simulink model "BEVplantModel"  (R2022b)
settings: Solver=daessc  StartTime=0  StopTime=50  RelTol=1e-3
PreLoadFcn:
  | % Load all parameters
  | BEVplantModelParam;
undefined symbols (not defined in the file): battery, cabin_T_init, coolant_pipe_D, coolant_valve_D_ratio_max, coolant_valve_D_ratio_min, coolant_valve_displacement, electricDrive, max_torque, vehicle, vehicleThermal
libraries: fl_lib x292, nesl_utility x67, SimscapeFluids_lib x15, ee_lib x11, sdl_lib x8, BatteryCurrentManagement x3, slpidlib x3, simulink x2, BatteryThermalManagement x1, autolibshared x1
(part 7 of 10)

== system BEVplantModel/Controller/BMS/MinMax Current Limiter/ODprotection ==
  Cur : Inport
  VoltMin : Inport  Port=2
  CellTpMax : Inport  Port=3
  CellTpMin : Inport  Port=4
  Add : Sum  Inputs=-+
  Constant : Constant  Value=10
  DchrgCurLim : Gain  Gain=battery.MaxDchrgCurLim
  DischCurrLimitMaxTp : Lookup_n-D  NumberOfTableDimensions=1  BreakpointsForDimension1=single([313, 318, 323, 333])  BreakpointsForDimension3=[5, 7]  Table=single([1, 0.5, 0.3, 0])  ExtrapMethod=Clip  UseLastTableValue=on  InternalRulePriority=Speed  RndMeth=Simplest
  DischCurrLimitMinTp : Lookup_n-D  NumberOfTableDimensions=1  BreakpointsForDimension1="single([263, 268,    273,   278, 283, 288, 293])"  BreakpointsForDimension3=[5, 7]  Table="single([0,  0.2, 0.3, 0.5, 0.75, 1, 1])"  ExtrapMethod=Clip  UseLastTableValue=on  InternalRulePriority=Speed  RndMeth=Simplest
  DischCurrLimitVolt : Lookup_n-D  NumberOfTableDimensions=1  BreakpointsForDimension1=single([2.5;3;3.5;4.2])  BreakpointsForDimension3=[5, 7]  Table=single([0 0.25 0.5 0.75])  ExtrapMethod=Clip  UseLastTableValue=on  InternalRulePriority=Speed  RndMeth=Simplest
  Gain : Gain  Gain=2
  Min : MinMax  Inputs=3
  Np_Module : Gain  Gain=battery.Np
  Relational Operator : RelationalOperator  Operator=<=  OutDataTypeStr=boolean  RndMeth=Simplest  InputSameDT=off
  DschCurLim : Outport
  ODWarn : Outport  Port=2
  tag scope: DschCurLim=global
  wires:
  Constant/1 -> Add/1
  Add/1 -> Relational Operator/1
  Relational Operator/1 -> ODWarn/1
  [DschCurLim] -> Add/2
  Cur/1 -> Relational Operator/2
  Min/1 -> DchrgCurLim/1
  DischCurrLimitMinTp/1 -> Min/3  "DischCurrLimMinTp"
  DischCurrLimitMaxTp/1 -> Min/2  "DischCurrLimMaxTp"
  CellTpMax/1 -> DischCurrLimitMaxTp/1
  Np_Module/1 -> [DschCurLim], Gain/1  "CurDchLmt"
  DchrgCurLim/1 -> Np_Module/1
  DischCurrLimitVolt/1 -> Min/1  "DischCurrLimVolt"
  VoltMin/1 -> DischCurrLimitVolt/1
  CellTpMin/1 -> DischCurrLimitMinTp/1
  Gain/1 -> DschCurLim/1  "CurDchLmt"

== system BEVplantModel/Controller/Range Estimator/Online Range/Energy Consumption ==
  V : Inport
  I : Inport  Port=2
  Constant : Constant  Value=3600
  Divide : Product  Inputs=*/
  Gain : Gain  Gain=-1
  Integrator : Integrator
  Product : Product
  E : Outport
  wires:
  Gain/1 -> Product/2
  Constant/1 -> Divide/2
  Integrator/1 -> Divide/1
  Product/1 -> Integrator/1
  I/1 -> Gain/1
  V/1 -> Product/1
  Divide/1 -> E/1

== system BEVplantModel/Controller/Range Estimator/Online Range/Subsystem ==
  E : Inport
  d : Inport  Port=2
  Add : Sum
  Constant2 : Constant
  Divide2 : Product  Inputs=*/
  E/D : Outport
  wires:
  Add/1 -> E/D/1
  Constant2/1 -> Add/2
  Divide2/1 -> Add/1
  d/1 -> Divide2/2
  E/1 -> Divide2/1

== system BEVplantModel/Controller/Thermal Control/Coolant Control/Battery Heater ==
  T_env : Inport
  T_coolant_battery_in : Inport  Port=2
  Constant : Constant  Value=0
  Relay : Relay  OnSwitchValue=15+273.15  OffSwitchValue=5+273.15  OnOutputValue=0  OffOutputValue=1  ZeroCross=off
  Switch : Switch  Criteria=u2 > Threshold  Threshold=5+273.15  SaturateOnIntegerOverflow=off  InputSameDT=off
  cmd_heater : Outport
  wires:
  Constant/1 -> Switch/1
  Relay/1 -> Switch/3
  T_env/1 -> Switch/2
  Switch/1 -> cmd_heater/1
  T_coolant_battery_in/1 -> Relay/1

== system BEVplantModel/Controller/Thermal Control/Coolant Control/Battery Pump ==
  cmd_motor_pump : Inport
  T_battery : Inport  Port=2
  cmd_chiller_bypass : Inport  Port=3
  parallel_serial : Inport  Port=4
  Constant : Constant  Value=0.3
  Constant1 : Constant  Value=0.5
  MinMax : MinMax  Function=max  Inputs=2
  Relay : Relay  OnSwitchValue=50+273.15  OffSwitchValue=45+273.15
  Switch : Switch  Criteria=u2 > Threshold  Threshold=0.5  SaturateOnIntegerOverflow=off  InputSameDT=off
  Switch1 : Switch  Criteria=u2 > Threshold  Threshold=0.5  SaturateOnIntegerOverflow=off  InputSameDT=off
  cmd_battery_pump : Outport
  wires:
  cmd_motor_pump/1 -> Switch/1
  MinMax/1 -> Switch/3
  Switch1/1 -> MinMax/2
  Relay/1 -> MinMax/1
  cmd_chiller_bypass/1 -> Switch1/2
  Constant1/1 -> Switch1/3
  Constant/1 -> Switch1/1
  Switch/1 -> cmd_battery_pump/1
  parallel_serial/1 -> Switch/2
  T_battery/1 -> Relay/1

== system BEVplantModel/Controller/Thermal Control/Coolant Control/Chiller Bypass ==
  T_battery : Inport
  Relay : Relay  OnSwitchValue=35+273.15  OffSwitchValue=30+273.15  OnOutputValue=0  OffOutputValue=1
  cmd_chiller_bypass : Outport
  wires:
  T_battery/1 -> Relay/1
  Relay/1 -> cmd_chiller_bypass/1

== system BEVplantModel/Controller/Thermal Control/Coolant Control/Motor Pump ==
  T_motor : Inport
  1-D Lookup Table : Lookup_n-D  NumberOfTableDimensions=1  BreakpointsForDimension1=[223.15 318.15 321.15 325.15 331.15 333.15 348.15 403.15]  IndexSearchMethod=Linear search  BeginIndexSearchUsingPreviousIndexResult=on  Table=[0 0 0.1 0.3 0.5 0.7 1 1]  InternalRulePriority=Speed  RndMeth=Simplest
  Saturation : Saturate  UpperLimit=1  LowerLimit=0.3
  cmd_motor_pump : Outport
  wires:
  Saturation/1 -> cmd_motor_pump/1
  1-D Lookup Table/1 -> Saturation/1
  T_motor/1 -> 1-D Lookup Table/1

== system BEVplantModel/Controller/Thermal Control/Coolant Control/Parallel-Serial Mode ==
  note: 0 = Parallel mode
      |
      | 1 = Serial mode
  cmd_chiller_bypass : Inport
  T_env : Inport  Port=2
  T_coolant_motor_out : Inport  Port=3
  Constant : Constant  Value=0
  MinMax : MinMax  Function=max  Inputs=2
  Relay : Relay  OnSwitchValue=35+273.15  OffSwitchValue=30+273.15  OnOutputValue=0  OffOutputValue=1
  Switch : Switch  Criteria=u2 > Threshold  Threshold=0.5  SaturateOnIntegerOverflow=off  InputSameDT=off
  cmd_parallel_serial : Outport
  wires:
  Relay/1 -> Switch/1
  cmd_chiller_bypass/1 -> Switch/2
  Switch/1 -> cmd_parallel_serial/1
  Constant/1 -> Switch/3
  MinMax/1 -> Relay/1
  T_coolant_motor_out/1 -> MinMax/2
  T_env/1 -> MinMax/1

== system BEVplantModel/Controller/Thermal Control/Coolant Control/Radiator Bypass ==
  T_coolant_motor_out : Inport
  Relay : Relay  OnSwitchValue=25+273.15  OffSwitchValue=20+273.15  OnOutputValue=0  OffOutputValue=1
  cmd_rad_bypass : Outport
  wires:
  T_coolant_motor_out/1 -> Relay/1
  Relay/1 -> cmd_rad_bypass/1

== system BEVplantModel/Controller/Thermal Control/Fan Control/Motor Requirement ==
  T_motor : Inport
  1-D Lookup Table : Lookup_n-D  NumberOfTableDimensions=1  BreakpointsForDimension1=[223.15 318.15 321.15 325.15 331.15 333.15 348.15 403.15]  IndexSearchMethod=Linear search  BeginIndexSearchUsingPreviousIndexResult=on  Table=[0 0 0.1 0.3 0.5 0.7 1 1]  InternalRulePriority=Speed  RndMeth=Simplest
  cmd_fan : Outport
  wires:
  1-D Lookup Table/1 -> cmd_fan/1
  T_motor/1 -> 1-D Lookup Table/1

== system BEVplantModel/Controller/Vehicle Control/Driver/Motor Speed Reference ==
  VehSpd : Inport  Unit=km/hr
  Constant1 : Constant  Value=vehicle.tireRollingRadius_cm
  Constant2 : Constant  Value=10/3
  Divide : Product  Inputs=*/
  Gain : Gain  Gain=2*pi
  Gain1 : Gain  Gain=1/100
  Product : Product
  Signal Specification : SignalSpecification  Unit=m/min
  Unit Conversion : UnitConversion
  MotorSpdRef : Outport  Unit=rpm  VectorParamsAs1DForOutWhenUnconnected=off
  wires:
  VehSpd/1 -> Unit Conversion/1
  Unit Conversion/1 -> Signal Specification/1
  Signal Specification/1 -> Divide/1
  Constant1/1 -> Gain1/1  "cm"
  Gain/1 -> Divide/2  "2*pi*R (m)"
  Divide/1 -> Product/1  "tireRpmRef"
  Constant2/1 -> Product/2
  Product/1 -> MotorSpdRef/1  "motorRpmRef"
  Gain1/1 -> Gain/1  "m"

== system BEVplantModel/Controller/Vehicle Control/Driver/Speed Controller ==
  Spd : Inport  Unit=rpm
      settings: AttributesFormatString=%<Unit>
  SpdRef : Inport  Port=2  Unit=rpm
      settings: AttributesFormatString=%<Unit>
  20Hz Lowpass Filter : TransferFcn  Denominator=[1/(2*pi*20) 1]
  Constant : Constant  Value=0
  GreaterThan : RelationalOperator  Operator=>  OutDataTypeStr=boolean  RndMeth=Simplest  InputSameDT=off
  Ki : Gain  Gain=5
  Kp : Gain  Gain=5
  Limits [-40,40] : Integrator  ExternalReset=rising  LimitOutput=on  UpperSaturationLimit=40  LowerSaturationLimit=-40  ZeroCross=off
  Saturation : Saturate  UpperLimit=vehicle.motorDrive.simplePmsmDrv_trqMax_Nm  LowerLimit=-vehicle.motorDrive.simplePmsmDrv_trqMax_Nm
      settings: AttributesFormatString=|
      | %<UpperLimit>
      | %<LowerLimit>
  Sum : Sum  Inputs=-+|
  Sum1 : Sum  Inputs=++|
  TrqPID : Outport  Unit=N*m  VectorParamsAs1DForOutWhenUnconnected=off
      settings: AttributesFormatString=%<Unit>
  wires:
  Saturation/1 -> TrqPID/1
  20Hz Lowpass Filter/1 -> GreaterThan/2, Sum/1
  Limits [-40,40]/1 -> Sum1/1
  Kp/1 -> Sum1/2
  Ki/1 -> Limits [-40,40]/1
  Sum/1 -> Kp/1, Ki/1
  Sum1/1 -> Saturation/1
  Spd/1 -> 20Hz Lowpass Filter/1
  SpdRef/1 -> Sum/2
  Constant/1 -> GreaterThan/1
  GreaterThan/1 -> Limits [-40,40]/2

== system BEVplantModel/Controller/Vehicle Control/Torque Control/Brake//Motor Trq Split ==
  note: Torque split between Break model and Modtor drive.
      | TrqCmdPID=Break torque + motor Torque
  TrqReq : Inport
  TrqLimit : Inport  Port=2
  BreakOn : Inport  Port=3
  Abs : Abs  ZeroCross=off  SaturateOnIntegerOverflow=off
  Braking Torque : Subsystem
  Bus Selector : BusSelector  OutputSignals=MaxChrgTrq,MaxDchTorque
  Constant : Constant  Value=vehicle.BrakeFactor
  Max1 : MinMax  Inputs=2  ZeroCross=off
  Switch : Switch  Criteria=u2 > Threshold  SaturateOnIntegerOverflow=off  InputSameDT=off
  TorqueCmd : Outport
  BrkTrq : Outport  Port=2
  wires:
  Bus Selector/2 -> Max1/1  "<MaxDchTorque>"
  TrqReq/1 -> Max1/2
  BreakOn/1 -> Switch/2
  Max1/1 -> Braking Torque/3(BrkTq), Switch/3
  TrqLimit/1 -> Bus Selector/1
  Braking Torque/1(MechBrkTq) -> Abs/1
  Braking Torque/2(RegenBrkTq) -> Switch/1
  Switch/1 -> TorqueCmd/1
  Abs/1 -> BrkTrq/1
  Bus Selector/1 -> Braking Torque/2(MaxChgTq)  "<MaxChrgTrq>"
  Constant/1 -> Braking Torque/1(BrkFac)

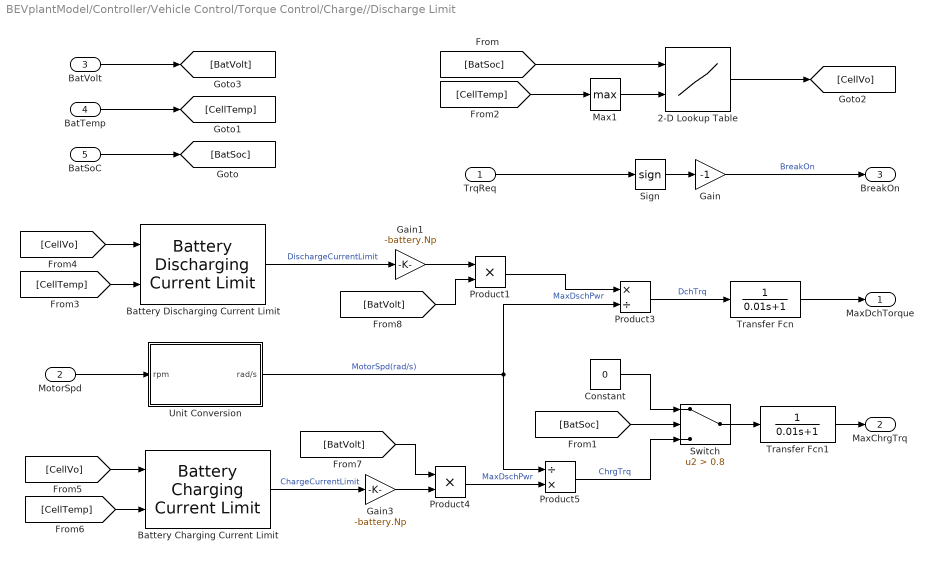
== system BEVplantModel/Controller/Vehicle Control/Torque Control/Charge//Discharge Limit ==
  TrqReq : Inport
  MotorSpd : Inport  Port=2
  BatVolt : Inport  Port=3
  BatTemp : Inport  Port=4
  BatSoC : Inport  Port=5
  2-D Lookup Table : Lookup_n-D  BreakpointsForDimension1=battery.SOC_vec  BreakpointsForDimension2=battery.T_vec  Table=battery.V0_mat  InternalRulePriority=Speed  RndMeth=Simplest
      settings: InputPortMap=u0,u1
  Battery Charging Current Limit : BatteryCurrentManagement/Battery Charging Current Limit  CellOvervoltageLimit=4.5  R0=0.0025  T_vec=[243.15, 258.15, 273.15, 288.15, 303.15, 318.15, 333.15]  CurrentLimitCoolestCell=[ 0, 0,0.5* battery.AH, battery.AH, battery.AH, battery.AH, battery.AH]  CurrentLimitHottestCell="[ battery.AH,  battery.AH,  battery.AH,  battery.AH,  battery.AH,  0.5*battery.AH, 0]"
      settings: LibrarySourceBlock=|
      | batt_sl_lib/Current Management/Battery Charging
      | Current Limit
  Battery Discharging Current Limit : BatteryCurrentManagement/Battery Discharging Current Limit  CellUndervoltageLimit=3  R0=0.0025  T_vec=[243.15, 258.15, 273.15, 288.15, 303.15, 318.15, 333.15]  CurrentLimitCoolestCell=[ 0, 0, battery.AH, 3*battery.AH, 3*battery.AH, 3*battery.AH, 3*battery.AH]  CurrentLimitHottestCell="[ 3*battery.AH,  3*battery.AH,  3*battery.AH,  3*battery.AH,  3*battery.AH,  battery.AH, 0]"
      settings: LibrarySourceBlock=|
      | batt_sl_lib/Current Management/Battery Discharging
      | Current Limit
  Constant : Constant  Value=0
  Gain : Gain  Gain=-1
  Gain1 : Gain  Gain=-battery.Np
  Gain3 : Gain  Gain=-battery.Np
  Max1 : MinMax  Function=max  ZeroCross=off
  Product1 : Product
  Product3 : Product  Inputs=*/
  Product4 : Product
  Product5 : Product  Inputs=/*
  Sign : Signum  ZeroCross=off
  Switch : Switch  Criteria=u2 > Threshold  Threshold=0.8  SaturateOnIntegerOverflow=off  InputSameDT=off
  Transfer Fcn : TransferFcn  Denominator=[0.01 1]
  Transfer Fcn1 : TransferFcn  Denominator=[0.01 1]
  Unit Conversion : Subsystem
  MaxDchTorque : Outport
  MaxChrgTrq : Outport  Port=2
  BreakOn : Outport  Port=3
  wires:
  Gain/1 -> BreakOn/1  "BreakOn"
  Product5/1 -> Switch/3  "ChrgTrq"
  TrqReq/1 -> Sign/1
  Sign/1 -> Gain/1
  Unit Conversion/1(rad/s) -> Product3/2, Product5/1  "MotorSpd(rad/s)"
  MotorSpd/1 -> Unit Conversion/1(rpm)
  [CellTemp] -> Battery Discharging Current Limit/2
  Product3/1 -> Transfer Fcn/1  "DchTrq"
  Battery Charging Current Limit/1 -> Gain3/1  "ChargeCurrentLimit"
  Gain3/1 -> Product4/2
  Product4/1 -> Product5/2  "MaxDschPwr"
  Gain1/1 -> Product1/1
  Transfer Fcn/1 -> MaxDchTorque/1
  Switch/1 -> Transfer Fcn1/1
  Max1/1 -> 2-D Lookup Table/2
  [CellVo] -> Battery Discharging Current Limit/1
  Battery Discharging Current Limit/1 -> Gain1/1  "DischargeCurrentLimit"
  [BatVolt] -> Product4/1
  [BatSoc] -> 2-D Lookup Table/1
  [BatSoc] -> Switch/2
  BatTemp/1 -> [CellTemp]
  [CellTemp] -> Max1/1
  2-D Lookup Table/1 -> [CellVo]
  [CellVo] -> Battery Charging Current Limit/1
  [CellTemp] -> Battery Charging Current Limit/2
  BatVolt/1 -> [BatVolt]
  [BatVolt] -> Product1/2
  Constant/1 -> Switch/1
  Transfer Fcn1/1 -> MaxChrgTrq/1
  Product1/1 -> Product3/1  "MaxDschPwr"
  BatSoC/1 -> [BatSoc]

== system BEVplantModel/Controller/Vehicle Control/Torque Control/Mech. Brake Model ==
  BreakOn : Inport
  BrkTrq : Inport  Port=2
  Brake Force (N) : Constant  Value=0
  Constant1 : Constant  Value=vehicle.tireRollingRadius_cm
  Gain : Gain  Gain=2*pi*4
  Gain1 : Gain  Gain=1/100
  Product : Product
  Switch : Switch  Criteria=u2 > Threshold  ZeroCross=off  SaturateOnIntegerOverflow=off  InputSameDT=off
  BrakeForce : Outport
  wires:
  Product/1 -> Switch/1  "BrakeForce"
  Constant1/1 -> Gain1/1  "cm"
  Gain/1 -> Product/1  "2*pi*R (m)"
  BrkTrq/1 -> Product/2
  BreakOn/1 -> Switch/2
  Brake Force (N)/1 -> Switch/3
  Gain1/1 -> Gain/1  "m"
  Switch/1 -> BrakeForce/1

== system BEVplantModel/Controller/Vehicle Control/Torque Control/Trq Split Fac ==
  Tq : Inport
  Stateflow : Stateflow chart  TreatAsAtomicUnit=on
  DrvMd : Outport
  TrqEM2fac : Outport  Port=2
  TrqEM1fac : Outport  Port=3
  wires:
  Tq/1 -> Stateflow/1(Tq)
  Stateflow/3(TrqEm1Fac) -> TrqEM1fac/1  "TrqEM1fac"
  Stateflow/2(TrqEm2Fac) -> TrqEM2fac/1  "TrqEM2fac"
  Stateflow/1(Mode) -> DrvMd/1  "DrvMd"

== system BEVplantModel/Vehicle/Chiller/Chiller Subsystem/Chiller Demand ==
  note: Chiller power Demand to current conversion
  No current : fl_lib/Physical Signals/Sources/PS Constant  constant=0 A
  PS Abs : fl_lib/Physical Signals/Nonlinear Operators/PS Abs
      settings: InternalSimscapePortConfiguration="{\"Bottom\":[],\"Left\":[{\"id\":\"I\",\"label\":\"\",\"type\":\"input\"}],\"Right\":[{\"id\":\"O\",\"label\":\"\",\"type\":\"output\"}],\"Top\":[]}"
  PS Abs1 : fl_lib/Physical Signals/Nonlinear Operators/PS Abs
      settings: InternalSimscapePortConfiguration="{\"Bottom\":[],\"Left\":[{\"id\":\"I\",\"label\":\"\",\"type\":\"input\"}],\"Right\":[{\"id\":\"O\",\"label\":\"\",\"type\":\"output\"}],\"Top\":[]}"
  PS Add : fl_lib/Physical Signals/Functions/PS Add
  PS Divide : fl_lib/Physical Signals/Functions/PS Divide
  PS Switch : fl_lib/Physical Signals/Nonlinear Operators/PS Switch  Threshold=0.5
      settings: InternalSimscapePortConfiguration="{\"Bottom\":[],\"Left\":[{\"id\":\"I1\",\"label\":\"\",\"type\":\"input\"},{\"id\":\"I2\",\"label\":\"\",\"type\":\"input\"},{\"id\":\"I3\",\"label\":\"\",\"type\":\"input\"}],\"Right\":[{\"id\":\"O\",\"label\":\"\",\"type\":\"output\"}],\"Top\":[]}"
  Zero Divide Protection : fl_lib/Physical Signals/Sources/PS Constant  constant=1 V
  Volt : PMIOPort  Side=Left
  BatSt : PMIOPort  Port=2  Side=Left
  P : PMIOPort  Port=3  Side=Left
  I : PMIOPort  Port=4  Side=Right
  connections:
  No current/RConn1 -- PS Switch/LConn3
  PS Add/LConn1 -- Volt/RConn1
  PS Switch/LConn1 -- PS Divide/RConn1
  BatSt/RConn1 -- PS Switch/LConn2
  I/RConn1 -- PS Abs1/RConn1
  PS Add/RConn1 -- PS Divide/LConn2
  PS Add/LConn2 -- Zero Divide Protection/RConn1
  PS Abs/RConn1 -- PS Divide/LConn1
  P/RConn1 -- PS Abs/LConn1
  PS Abs1/LConn1 -- PS Switch/RConn1

== system BEVplantModel/Vehicle/Front Motor (EM1)/Emotor/Air HTC calculation ==
  Rotor Taylor Couette  HTC : Subsystem
  Rotor side  HTC : Subsystem
  w : PMIOPort  Side=Left
  HTC_TC : PMIOPort  Port=2  Side=Right
  HTC : PMIOPort  Port=3  Side=Right
  connections:
  Rotor side  HTC/LConn1 -- w/RConn1 -- Rotor Taylor Couette  HTC/LConn1
  HTC/RConn1 -- Rotor side  HTC/RConn1
  Rotor Taylor Couette  HTC/RConn1 -- HTC_TC/RConn1

== system BEVplantModel/Vehicle/Front Motor (EM1)/Emotor/Loss Estimation0 ==
  "Copper Loss " : Subsystem
  Iron Loss : Subsystem
  Subsystem : Subsystem
  Hmot : PMIOPort  Side=Left
  I2R : PMIOPort  Port=2  Side=Right
  H_rt : PMIOPort  Port=3  Side=Right
  H_st : PMIOPort  Port=4  Side=Right
  Current : PMIOPort  Port=5  Side=Left
  connections:
  H_rt/RConn1 -- Iron Loss/RConn1
  Iron Loss/RConn2 -- H_st/RConn1
  Hmot/RConn1 -- Subsystem/LConn1
  "Copper Loss "/LConn1 -- Current/RConn1
  "Copper Loss "/RConn1 -- Iron Loss/LConn2 -- I2R/RConn1
  Subsystem/RConn1 -- Iron Loss/LConn1

== system BEVplantModel/Vehicle/Front Motor (EM1)/Emotor/Sensing Ref Torque ==
  " " : Inport
  Simulink-PS G1 : nesl_utility/Simulink-PS Converter  PhysicalDomain=network_engine_domain  SubClassName=ps_input  LeftPortType=input  RightPortType=output  PseudoPeriodic=off  Frequencies=[]  NoiseDistribution=none  NoiseParameters=[]  Unit=N*m  AffineConversion=off  FilteringAndDerivatives=zero  SimscapeFilterOrder=1  InputFilterTimeConstant=1e-6  UdotUserProvided=1
  "  " : PMIOPort  Side=Right
  wires:
  " "/1 -> Simulink-PS G1/1
  connections:
  Simulink-PS G1/RConn1 -- "  "/RConn1

== system BEVplantModel/Vehicle/Front Motor (EM1)/Emotor/Sensing wMotor ==
  PS-Simulink Converter : nesl_utility/PS-Simulink Converter  PhysicalDomain=network_engine_domain  SubClassName=ps_output  LeftPortType=input  RightPortType=output  PseudoPeriodic=off  Frequencies=[]  VectorFormat=1-D array  Unit=rpm  AffineConversion=off
  PS : PMIOPort  Side=Left
  SL : Outport  VectorParamsAs1DForOutWhenUnconnected=off
  wires:
  PS-Simulink Converter/1 -> SL/1
  connections:
  PS/RConn1 -- PS-Simulink Converter/LConn1

== system BEVplantModel/Vehicle/Front Motor (EM1)/Emotor/Speed Measurement ==
  Ideal Rotational Motion Sensor : fl_lib/Mechanical/Mechanical Sensors/Ideal Rotational Motion Sensor  reference=foundation.enum.MeasurementReference.difference  acceleration_port=false  velocity_port=true  position_port=true  wrap_angle=false  offset=0 rad
  MRRef1 : fl_lib/Mechanical/Rotational Elements/Mechanical Rotational Reference
  spd : PMIOPort  Side=Right
  mot : PMIOPort  Port=2  Side=Left
  connections:
  MRRef1/LConn1 -- Ideal Rotational Motion Sensor/RConn1
  mot/RConn1 -- Ideal Rotational Motion Sensor/LConn1
  spd/RConn1 -- Ideal Rotational Motion Sensor/RConn2

== system BEVplantModel/Vehicle/Front Motor (EM1)/Emotor/Temperature ==
  Rotor Thermal Block : Subsystem
  Stator Thermal Block : Subsystem
  I2R : PMIOPort  Side=Left
  H_rt : PMIOPort  Port=2  Side=Left
  H_st : PMIOPort  Port=3  Side=Left
  HTC_TC : PMIOPort  Port=4  Side=Left
  HTC : PMIOPort  Port=5  Side=Left
  Tc : PMIOPort  Port=6  Side=Right
  Tm : PMIOPort  Port=7  Side=Right
  H : PMIOPort  Port=8  Side=Right
  connections:
  H/RConn1 -- Stator Thermal Block/LConn1
  H_rt/RConn1 -- Rotor Thermal Block/RConn1
  H_st/RConn1 -- Stator Thermal Block/RConn1
  I2R/RConn1 -- Stator Thermal Block/RConn2
  HTC_TC/RConn1 -- Rotor Thermal Block/RConn2
  HTC/RConn1 -- Rotor Thermal Block/RConn3
  Tm/RConn1 -- Rotor Thermal Block/LConn1
  Tc/RConn1 -- Stator Thermal Block/LConn2

== system BEVplantModel/Vehicle/Front Motor (EM1)/Emotor/current sensing1 ==
  Current Sensor : fl_lib/Electrical/Electrical Sensors/Current Sensor
  " " : PMIOPort  Side=Left
  "  " : PMIOPort  Port=2  Side=Right
  "  I" : PMIOPort  Port=3  Side=Right
  connections:
  Current Sensor/RConn2 -- "  "/RConn1
  Current Sensor/LConn1 -- " "/RConn1
  Current Sensor/RConn1 -- "  I"/RConn1

== system BEVplantModel/Vehicle/Front Motor (EM1)/Inverter Power Module Thermal/PM Cauer thermall ==
  Casing mass : fl_lib/Thermal/Thermal Elements/Thermal Mass  mass=0.5 kg  sp_heat=447 J/(K*kg)  num_ports=foundation.enum.numPorts2.one  T_specify=on  T_priority=High  T=vehicleThermal.coolant_T_init K  T_nominal_specify=off  T_nominal_unit=K  T_nominal_value=1  Q_specify=off  Q_priority=None  Q=0 W  Q_nominal_specify=off  Q_nominal_unit=W  Q_nominal_value=1
  Conductive Heat Transfer : fl_lib/Thermal/Thermal Elements/Conductive Heat Transfer  thermal_type=foundation.enum.ConstantVariableTabulated.Constant  wall_geometry=foundation.enum.ConductionWallGeometry.Planar  area=1e-4 m^2  thickness=0.1 m  d_in=0.05 m  d_out=0.1 m  L=1 m  th_cond_min=10 W/(K*m)  th_cond=401 W/(K*m)  th_cond_TLU=[413, 401, 392, 383, 371, 357, 342] W/(K*m)  temp_TLU=[200, 273, 400, 600, 800, 1000, 1200] K  T_specify=off  T_priority=None  T=0 K  T_nominal_specify=off  T_nominal_unit=K  T_nominal_value=1  Q_specify=off  Q_priority=None  Q=0 W  Q_nominal_specify=off  Q_nominal_unit=W  Q_nominal_value=1
  Controlled Heat Flow Rate Source : fl_lib/Thermal/Thermal Sources/Controlled Heat Flow Rate Source
  Controlled Heat Flow Rate Source1 : fl_lib/Thermal/Thermal Sources/Controlled Heat Flow Rate Source
  Heatsink : ee_lib/Passive/Thermal/Heatsink  parameterization=ee.enum.passive.thermal.heatsinkParam.rectangularFin  convection=ee.enum.passive.thermal.heatsinkConvection.specifyFlowSpeed  T_vec_Q=[10, 30, 50, 70, 90] K  v_vec_Q=[0, 1, 2, 3] m/s  Q_TLU1=[6.1, 23.6, 44.5, 67.5, 92.3] W  Q_TLU2=[6.1, 18.8, 22.8, 25.7; 23.6, 61.1, 73, 81.5; 44.5, 106.4, 125.9, 140.1; 67.5, 153.5, 180.7, 200.3; 92.3, 202.1, 236.9, 262] W  T_vec_h=[10, 30, 50, 70, 90] K  v_vec_h=[0, 1, 2, 3] m/s  h_TLU1=[5.4, 7.02, 7.98, 8.68, 9.26] W/(K*m^2)  h_TLU2=[5.4, 17.86, 22.17, 25.41; 7.02, 19.49, 23.8, 27.03; 7.97, 20.44, 24.75, 27.99; 8.68, 21.15, 25.46, 28.69; 9.26, 21.73, 26.04, 29.27] W/(K*m^2)  h_vec=[5, 10, 15, 20, 25, 30] W/(K*m^2)  eff_TLU=[96.97, 94.16, 91.53, 89.08, 86.78, 84.62]  height=electricDrive.HeatsinkParams.Height m  thick=electricDrive.HeatsinkParams.Thick m  depth=electricDrive.HeatsinkParams.Depth m  gap=electricDrive.HeatsinkParams.Gap m  num_fins=electricDrive.HeatsinkParams.NumFins  k_fin=386 W/(K*m)  A_total=0.1171 m^2  nu=2.62e-6 m^2/s  alpha=6.55e-8 m^2/s  k_fluid=0.55 W/(K*m)  beta=5.82e-4 1/K  mass=electricDrive.HeatsinkParams.Mass kg  sp_heat=437 J/(K*kg)  T_hs_specify=on  T_hs_priority=High  T_hs=vehicleThermal.coolant_T_init K  T_hs_nominal_specify=off  T_hs_nominal_unit=K  T_hs_nominal_value=1  Q_A_specify=off  Q_A_priority=None  Q_A=0 W  Q_A_nominal_specify=on  Q_A_nominal_unit=W  Q_A_nominal_value=1  Q_C_specify=off  Q_C_priority=None  Q_C=0 W  Q_C_nominal_specify=on  Q_C_nominal_unit=W  Q_C_nominal_value=1
      settings: InternalSimscapePortConfiguration="{\"Bottom\":[{\"id\":\"C\",\"label\":\"C\",\"type\":\"foundation.thermal.thermal\"}],\"Left\":[{\"id\":\"v\",\"label\":\"v\",\"type\":\"input\"}],\"Right\":[],\"Top\":[{\"id\":\"A\",\"label\":\"A\",\"type\":\"foundation.thermal.thermal\"}]}"
  Probe : SimscapeProbe  BoundBlock=6711  Variables={Tvec}
  Probe1 : SimscapeProbe  BoundBlock=6712  Variables={Tvec}
  Selector : Selector  InputPortWidth=4  IndexOptions=Index vector (dialog)  Indices=[1]  OutputSizes=1
  Selector1 : Selector  InputPortWidth=4  IndexOptions=Index vector (dialog)  Indices=[1]  OutputSizes=1
  Thermal Reference : fl_lib/Thermal/Thermal Elements/Thermal Reference
  Thermal Reference1 : fl_lib/Thermal/Thermal Elements/Thermal Reference
  Thermal Resistor : ee_lib/Passive/Thermal/Thermal Resistor  R=1e-3 K/W  T_specify=off  T_priority=None  T=0 K  T_nominal_specify=off  T_nominal_unit=K  T_nominal_value=1  Q_specify=off  Q_priority=None  Q=0 W  Q_nominal_specify=off  Q_nominal_unit=W  Q_nominal_value=1
      settings: InternalSimscapePortConfiguration="{\"Bottom\":[],\"Left\":[{\"id\":\"A\",\"label\":\"A\",\"type\":\"foundation.thermal.thermal\"}],\"Right\":[{\"id\":\"B\",\"label\":\"B\",\"type\":\"foundation.thermal.thermal\"}],\"Top\":[]}"
  ThermalModel_BodyDiode_6LumpedIn : ee_lib/Passive/Thermal/Cauer Thermal Model  parameterize_foster=true  resistance_data=1e-3 * [2.6468, 3.8701, 1.2007, .8824] K/W  tau_data=[.0086, .054, .3624, 1.651] s  resistance_data_foster=electricDrive.PMparams.RthDiode K/W  tau_data_foster=electricDrive.PMparams.tauthDiode s  refPort=simscape.enum.onoff.off  Tvec_specify=on  Tvec_priority=High  Tvec=electricDrive.PMparams.TinitDiode K  Tvec_nominal_specify=off  Tvec_nominal_unit=K  Tvec_nominal_value=1  Q_A_specify=off  Q_A_priority=None  Q_A=0 W  Q_A_nominal_specify=off  Q_A_nominal_unit=W  Q_A_nominal_value=1  Q_B_specify=off  Q_B_priority=None  Q_B=0 W  Q_B_nominal_specify=off  Q_B_nominal_unit=W  Q_B_nominal_value=1
      settings: InternalSimscapePortConfiguration="{\"Bottom\":[],\"Left\":[{\"id\":\"A\",\"label\":\"A\",\"type\":\"foundation.thermal.thermal\"}],\"Right\":[{\"id\":\"B\",\"label\":\"B\",\"type\":\"foundation.thermal.thermal\"}],\"Top\":[]}"
  ThermalModel_IGBT_6LumpedIn : ee_lib/Passive/Thermal/Cauer Thermal Model  parameterize_foster=true  resistance_data=1e-3 * [2.6468, 3.8701, 1.2007, .8824] K/W  tau_data=[.0086, .054, .3624, 1.651] s  resistance_data_foster=electricDrive.PMparams.RthIGBT K/W  tau_data_foster=electricDrive.PMparams.tauthIGBT s  refPort=simscape.enum.onoff.off  Tvec_specify=on  Tvec_priority=High  Tvec=electricDrive.PMparams.TinitIGBT K  Tvec_nominal_specify=off  Tvec_nominal_unit=K  Tvec_nominal_value=1  Q_A_specify=off  Q_A_priority=None  Q_A=0 W  Q_A_nominal_specify=off  Q_A_nominal_unit=W  Q_A_nominal_value=1  Q_B_specify=off  Q_B_priority=None  Q_B=0 W  Q_B_nominal_specify=off  Q_B_nominal_unit=W  Q_B_nominal_value=1
      settings: InternalSimscapePortConfiguration="{\"Bottom\":[],\"Left\":[{\"id\":\"A\",\"label\":\"A\",\"type\":\"foundation.thermal.thermal\"}],\"Right\":[{\"id\":\"B\",\"label\":\"B\",\"type\":\"foundation.thermal.thermal\"}],\"Top\":[]}"
  Unit Delay1 : UnitDelay  SampleTime=-1  HasFrameUpgradeWarning=on
  Unit Delay2 : UnitDelay  SampleTime=-1  HasFrameUpgradeWarning=on
  Inverter Heat : PMIOPort  Side=Left
  Averaged Diode Loss : PMIOPort  Port=2  Side=Right
  Averaged IGBT Loss : PMIOPort  Port=3  Side=Right
  Coolant Speed : PMIOPort  Port=4  Side=Right
  IGBT : Outport
  Diode : Outport  Port=2
  wires:
  Probe/1 -> Selector1/1
  Probe1/1 -> Selector/1
  Unit Delay2/1 -> IGBT/1
  Unit Delay1/1 -> Diode/1
  Selector/1 -> Unit Delay2/1
  Selector1/1 -> Unit Delay1/1
  connections:
  Thermal Resistor/RConn1 -- Controlled Heat Flow Rate Source1/LConn1 -- ThermalModel_BodyDiode_6LumpedIn/LConn1
  Thermal Reference/LConn1 -- Controlled Heat Flow Rate Source/RConn2
  Controlled Heat Flow Rate Source/LConn1 -- ThermalModel_IGBT_6LumpedIn/LConn1 -- Thermal Resistor/LConn1
  Controlled Heat Flow Rate Source1/RConn1 -- Averaged Diode Loss/RConn1
  ThermalModel_BodyDiode_6LumpedIn/RConn1 -- ThermalModel_IGBT_6LumpedIn/RConn1 -- Conductive Heat Transfer/LConn1
  Conductive Heat Transfer/RConn1 -- Casing mass/LConn1 -- Heatsink/RConn1
  Thermal Reference1/LConn1 -- Controlled Heat Flow Rate Source1/RConn2
  Controlled Heat Flow Rate Source/RConn1 -- Averaged IGBT Loss/RConn1
  Inverter Heat/RConn1 -- Heatsink/LConn2
  Heatsink/LConn1 -- Coolant Speed/RConn1

== system BEVplantModel/Vehicle/HVAC/Cabin/HVAC Control ==
  Tenv : Inport
  Tptc : Inport  Port=2
  Tcabin : Inport  Port=3
  TacVent : Inport  Port=4
  Tsetpoint : Inport  Port=5
  acOnOff : Inport  Port=6
  Cabin Air Control : Subsystem
  cmdBlower : Outport
  PTC : Outport  Port=2
  cmdCool : Outport  Port=3
  wires:
  Cabin Air Control/2(cmdPTC) -> PTC/1
  Tptc/1 -> Cabin Air Control/4(Tptc)
  Tenv/1 -> Cabin Air Control/3(Tenv)
  Tsetpoint/1 -> Cabin Air Control/2(Tsetpoint)
  Cabin Air Control/1(cmdBlower) -> cmdBlower/1
  Tcabin/1 -> Cabin Air Control/1(Tcabin)
  Cabin Air Control/3(cmdCool) -> cmdCool/1
  TacVent/1 -> Cabin Air Control/5(TacVent)
  acOnOff/1 -> Cabin Air Control/6(acOnOff)

== system BEVplantModel/Vehicle/HVAC/Cabin/HVAC Plant ==
  EnvTp : Inport
  cmdBlower : Inport  Port=2
  cmdPTC : Inport  Port=3
  cmdCool : Inport  Port=4
  Blower : Subsystem  Tag=PublishSubsystem
      settings: PortSchema="{\"entries\":[{\"content\":{\"sides\":[{\"content\":{\"connectorIds\":[]},\"type\":\"ConnectorPlacement.EquallySpacedRectSide\",\"uuid\":\"e68f4e4f-d2a0-4f21-a3dd-a8ccea0ce87c\"},{\"content\":{\"connectorIds\":[\"In1\"],\"side\":\"RIGHT\"},\"type\":\"ConnectorPlacement.EquallySpacedRectSide\",\"uuid\":\"01f15736-e6d7-4b17-9e84-cef8e8356dfe\"},{\"content\":{\"connectorIds\":[\"LConn1\"],\"side\":\"TOP\"},\"type\":\"ConnectorPlacement.EquallySpacedRectSide\",\"uuid\":\"cb1790c7-7993-46e4-a971-f0b801f1d2ca\"},{\"content\":{\"connectorIds\":[\"RConn1\"],\"side\":\"BOTTOM\"},\"type\":\"ConnectorPlacement.EquallySpacedRectSide\",\"uuid\":\"4227c4aa-9146-4cfe-9198-d14a991805e7\"},{\"content\":{\"connectorIds\":[],\"side\":\"HIDDEN\"},\"type\":\"ConnectorPlacement.EquallySpacedRectSide\",\"uuid\":\"e2e3575c-3b20-453d-a897-62a34bc693b5\"}]},\"type\":\"ConnectorPlacement.EquallySpacedConnector\",\"uuid\":\"0a7b2bb7-4c38-48ec-bfc1-fef0f38ff266\"}],\"packageUris\":[\"http://schema.mathworks.com/mf0/Connector/R2020b\"],\"version\":\"1.0\"}"
      mask Display:
      | plot(100*cos(linspace(0, 2*pi, 500)), 100*sin(linspace(0, 2*pi, 500)))
      | plot([28 80], [96 -60])
      | plot([-28 -80], [96 -60])
      | patch(-50*sin(3*linspace(0, pi, 500)).*cos(linspace(0, pi, 500)), -50*sin(3*linspace(0, pi, 500)).*sin(linspace(0, pi, 500)), [0 0 0])
  Cabin Air Volume : fl_lib/Moist Air/Elements/Constant Volume Chamber (MA)  volume=3 m^3  num_ports=foundation.enum.num_ports.two  area_A=vehicleThermal.cabin_duct_area m^2  area_B=vehicleThermal.cabin_duct_area m^2  area_C=0.01 m^2  area_D=0.01 m^2  RH_ws=1  time_constant=1e-3 s  moisture_trace_gas_source=foundation.enum.moisture_trace_gas_source.none  moisture_source_spec=foundation.enum.moisture_source_spec.vapor  moisture_mass_flow=0 kg/s  moisture_temperature_spec=foundation.enum.temperature_spec.atmospheric  moisture_temperature=293.15 K  trace_gas_mass_flow=0 kg/s  trace_gas_temperature_spec=foundation.enum.temperature_spec.atmospheric  trace_gas_temperature=293.15 K  p_I_specify=on  p_I_priority=High  p_I=vehicleThermal.cabin_p_init MPa  p_I_nominal_specify=off  p_I_nominal_unit=MPa  p_I_nominal_value=1  T_I_specify=on  T_I_priority=High  T_I=vehicleThermal.cabin_T_init K  T_I_nominal_specify=off  T_I_nominal_unit=K  T_I_nominal_value=1  RH_I_specify=on  RH_I_priority=High  RH_I=vehicleThermal.cabin_RH_init  RH_I_nominal_specify=off  RH_I_nominal_unit=1  RH_I_nominal_value=1  x_w_I_specify=off  x_w_I_priority=None  x_w_I=0  x_w_I_nominal_specify=off  x_w_I_nominal_unit=1  x_w_I_nominal_value=1  y_w_I_specify=off  y_w_I_priority=None  y_w_I=0  y_w_I_nominal_specify=off  y_w_I_nominal_unit=1  y_w_I_nominal_value=1  HR_I_specify=off  HR_I_priority=None  HR_I=0  HR_I_nominal_specify=off  HR_I_nominal_unit=1  HR_I_nominal_value=1  x_g_I_specify=off  x_g_I_priority=High  x_g_I=0  x_g_I_nominal_specify=off  x_g_I_nominal_unit=1  x_g_I_nominal_value=1  y_g_I_specify=off  y_g_I_priority=None  y_g_I=0  y_g_I_nominal_specify=off  y_g_I_nominal_unit=1  y_g_I_nominal_value=1
      settings: InternalSimscapePortConfiguration="{\"Bottom\":[],\"Left\":[{\"id\":\"A\",\"label\":\"A\",\"type\":\"foundation.moist_air.moist_air\"},{\"id\":\"B\",\"label\":\"B\",\"type\":\"foundation.moist_air.moist_air\"}],\"Right\":[{\"id\":\"W\",\"label\":\"W\",\"type\":\"output\"},{\"id\":\"F\",\"label\":\"F\",\"type\":\"output\"},{\"id\":\"H\",\"label\":\"H\",\"type\":\"foundation.thermal.thermal\"}],\"Top\":[]}"
  Cabin Heat Transfer : Subsystem  Tag=PublishSubsystem  mask(Cabin Heat Transfer){glass_area=3.5, glass_thickness=0.004, glass_mass=3.5 * 0.004 * 2600, glass_specific_heat=840, glass_conductivity=0.96, glass_heat_coeff=40, glass_initial_temperature=vehicleThermal.ambient, doors_area=4, doors_thickness=0.06, doors_mass=75, doors_specific_heat=500, doors_conductivity=0.08, doors_heat_coeff=40, doors_initial_temperature=vehicleThermal.ambient, roof_area=2, roof_thickness=0.04, roof_mass=30, roof_specific_heat=500, roof_conductivity=0.08, roof_heat_coeff=40, roof_initial_temperature=vehicleThermal.ambient}
      mask prompts: glass_area "Area (m^2)"; glass_thickness "Thickness (m)"; glass_mass "Mass (kg)"; glass_specific_heat "Specific heat (J/kg/K)"; glass_conductivity "Thermal conductivity (W/m/K)"; glass_heat_coeff "Convective heat transfer coefficient (W/m^2/K)"; glass_initial_temperature "Initial temperature (degC)"; doors_area "Area (m^2)"; doors_thickness "Thickness (m)"; doors_mass "Mass (kg)"; doors_specific_heat "Specific heat (J/kg/K)"; doors_conductivity "Thermal conductivity (W/m/K)"; doors_heat_coeff "Convective heat transfer coefficient (W/m^2/K)"; doors_initial_temperature "Initial temperature (degC)"; roof_area "Area (m^2)"; roof_thickness "Thickness (m)"; roof_mass "Mass (kg)"; roof_specific_heat "Specific heat (J/kg/K)"; roof_conductivity "Thermal conductivity (W/m/K)"; roof_heat_coeff "Convective heat transfer coefficient (W/m^2/K)"; roof_initial_temperature "Initial temperature (degC)"
      mask DialogControl GlassTabVar Prompt: Glass
      mask DialogControl DoorsTabVar Prompt: Doors
      mask DialogControl RoofTabVar Prompt: Roof
  CabinTp degC : Display
  Cooler : Subsystem
      settings: PortSchema="{\"entries\":[{\"content\":{\"sides\":[{\"content\":{\"connectorIds\":[\"In1\"]},\"type\":\"ConnectorPlacement.EquallySpacedRectSide\",\"uuid\":\"60def91b-13e6-4480-ae56-52c2c285a8b5\"},{\"content\":{\"connectorIds\":[\"Out1\"],\"side\":\"RIGHT\"},\"type\":\"ConnectorPlacement.EquallySpacedRectSide\",\"uuid\":\"3b6e461f-de22-4d5d-9340-a11e5b08e122\"},{\"content\":{\"connectorIds\":[\"LConn1\"],\"side\":\"TOP\"},\"type\":\"ConnectorPlacement.EquallySpacedRectSide\",\"uuid\":\"435062c2-883f-48fc-85e7-b5ad994d9104\"},{\"content\":{\"connectorIds\":[\"RConn1\"],\"side\":\"BOTTOM\"},\"type\":\"ConnectorPlacement.EquallySpacedRectSide\",\"uuid\":\"b78e2a7c-b7f6-462e-adbf-ed5741c86226\"}]},\"type\":\"ConnectorPlacement.EquallySpacedConnector\",\"uuid\":\"60d5b249-3c20-4d45-b0b7-63dc51f9d167\"}],\"packageUris\":[\"http://schema.mathworks.com/mf0/Connector/R2020b\"],\"version\":\"1.0\"}"
      mask Display: disp(get_param(gcb, 'Name'))
  Environment Temperature : fl_lib/Thermal/Thermal Sources/Controlled Temperature Source
  K to degC : Subsystem
  Measurement Selector (MA) : fl_lib/Moist Air/Sensors/Measurement Selector (MA)  moisture_spec=foundation.enum.moisture_spec.relative_humidity  trace_gas_spec=foundation.enum.trace_gas_spec.mass_fraction
  PS-Simulink Converter1 : nesl_utility/PS-Simulink Converter  PhysicalDomain=network_engine_domain  SubClassName=ps_output  LeftPortType=input  RightPortType=output  PseudoPeriodic=off  Frequencies=[]  VectorFormat=1-D array  Unit=K  AffineConversion=on
  PTC : Subsystem
      settings: PortSchema="{\"entries\":[{\"content\":{\"sides\":[{\"content\":{\"connectorIds\":[\"In1\"]},\"type\":\"ConnectorPlacement.EquallySpacedRectSide\",\"uuid\":\"60def91b-13e6-4480-ae56-52c2c285a8b5\"},{\"content\":{\"connectorIds\":[\"RConn1\",\"Out1\"],\"side\":\"RIGHT\"},\"type\":\"ConnectorPlacement.EquallySpacedRectSide\",\"uuid\":\"3b6e461f-de22-4d5d-9340-a11e5b08e122\"},{\"content\":{\"connectorIds\":[\"LConn1\"],\"side\":\"TOP\"},\"type\":\"ConnectorPlacement.EquallySpacedRectSide\",\"uuid\":\"435062c2-883f-48fc-85e7-b5ad994d9104\"}]},\"type\":\"ConnectorPlacement.EquallySpacedConnector\",\"uuid\":\"60d5b249-3c20-4d45-b0b7-63dc51f9d167\"}],\"packageUris\":[\"http://schema.mathworks.com/mf0/Connector/R2020b\"],\"version\":\"1.0\"}"
      mask Display: disp(get_param(gcb, 'Name'))
  Simulink-PS Converter : nesl_utility/Simulink-PS Converter  PhysicalDomain=network_engine_domain  SubClassName=ps_input  LeftPortType=input  RightPortType=output  PseudoPeriodic=off  Frequencies=[]  NoiseDistribution=none  NoiseParameters=[]  Unit=K  AffineConversion=on  FilteringAndDerivatives=provide  SimscapeFilterOrder=1  InputFilterTimeConstant=0.001  UdotUserProvided=0
  Thermal Reference1 : fl_lib/Thermal/Thermal Elements/Thermal Reference
  ptcTp : Outport
  CoolerTp : Outport  Port=2
  cabinTp : Outport  Port=3
  wires:
  EnvTp/1 -> Simulink-PS Converter/1
  cmdPTC/1 -> PTC/1(cmd)
  cmdBlower/1 -> Blower/1(cmd_blower)
  cmdCool/1 -> Cooler/1(cmd)
  PS-Simulink Converter1/1 -> K to degC/1(" "), cabinTp/1  "CabinTp"
  PTC/1(T) -> ptcTp/1
  Cooler/1(T) -> CoolerTp/1
  K to degC/1("  ") -> CabinTp degC/1
  connections:
  Environment Temperature/RConn1 -- Simulink-PS Converter/RConn1
  Environment Temperature/LConn1 -- Cabin Heat Transfer/RConn1
  Blower/RConn1 -- Cabin Air Volume/LConn1
  Cabin Air Volume/LConn2 -- PTC/RConn1
  Cabin Air Volume/RConn3 -- Cabin Heat Transfer/LConn1
  Thermal Reference1/LConn1 -- Environment Temperature/RConn2
  Measurement Selector (MA)/LConn1 -- Cabin Air Volume/RConn2
  Cooler/RConn1 -- PTC/LConn1
  Measurement Selector (MA)/RConn2 -- PS-Simulink Converter1/LConn1
  Blower/LConn1 -- Cooler/LConn1

== system BEVplantModel/Vehicle/Heater/Heater Subsystem/Heater Demand ==
  note: Heater power Demand to current conversion
  No current : fl_lib/Physical Signals/Sources/PS Constant  constant=0 A
  PS Abs1 : fl_lib/Physical Signals/Nonlinear Operators/PS Abs
      settings: InternalSimscapePortConfiguration="{\"Bottom\":[],\"Left\":[{\"id\":\"I\",\"label\":\"\",\"type\":\"input\"}],\"Right\":[{\"id\":\"O\",\"label\":\"\",\"type\":\"output\"}],\"Top\":[]}"
  PS Add : fl_lib/Physical Signals/Functions/PS Add
  PS Divide : fl_lib/Physical Signals/Functions/PS Divide
  PS Switch : fl_lib/Physical Signals/Nonlinear Operators/PS Switch  Threshold=0.5
      settings: InternalSimscapePortConfiguration="{\"Bottom\":[],\"Left\":[{\"id\":\"I1\",\"label\":\"\",\"type\":\"input\"},{\"id\":\"I2\",\"label\":\"\",\"type\":\"input\"},{\"id\":\"I3\",\"label\":\"\",\"type\":\"input\"}],\"Right\":[{\"id\":\"O\",\"label\":\"\",\"type\":\"output\"}],\"Top\":[]}"
  Zero Divide Protection : fl_lib/Physical Signals/Sources/PS Constant  constant=1 V
  Volt : PMIOPort  Side=Left
  BatSt : PMIOPort  Port=2  Side=Left
  P : PMIOPort  Port=3  Side=Left
  I : PMIOPort  Port=4  Side=Right
  connections:
  No current/RConn1 -- PS Switch/LConn3
  PS Add/LConn1 -- Volt/RConn1
  PS Switch/LConn1 -- PS Divide/RConn1
  BatSt/RConn1 -- PS Switch/LConn2
  I/RConn1 -- PS Abs1/RConn1
  PS Add/RConn1 -- PS Divide/LConn2
  PS Add/LConn2 -- Zero Divide Protection/RConn1
  P/RConn1 -- PS Divide/LConn1
  PS Abs1/LConn1 -- PS Switch/RConn1

== system BEVplantModel/Vehicle/Rear Motor (EM2)/Emotor/Air HTC calculation ==
  Rotor Taylor Couette  HTC : Subsystem
  Rotor side  HTC : Subsystem
  w : PMIOPort  Side=Left
  HTC_TC : PMIOPort  Port=2  Side=Right
  HTC : PMIOPort  Port=3  Side=Right
  connections:
  Rotor side  HTC/LConn1 -- w/RConn1 -- Rotor Taylor Couette  HTC/LConn1
  HTC/RConn1 -- Rotor side  HTC/RConn1
  Rotor Taylor Couette  HTC/RConn1 -- HTC_TC/RConn1

== system BEVplantModel/Vehicle/Rear Motor (EM2)/Emotor/Loss Estimation ==
  "Copper Loss " : Subsystem
  Iron Loss : Subsystem
  Subsystem : Subsystem
  Hmot : PMIOPort  Side=Left
  I2R : PMIOPort  Port=2  Side=Right
  H_rt : PMIOPort  Port=3  Side=Right
  H_st : PMIOPort  Port=4  Side=Right
  Current : PMIOPort  Port=5  Side=Left
  connections:
  H_rt/RConn1 -- Iron Loss/RConn1
  Iron Loss/RConn2 -- H_st/RConn1
  Hmot/RConn1 -- Subsystem/LConn1
  "Copper Loss "/LConn1 -- Current/RConn1
  "Copper Loss "/RConn1 -- Iron Loss/LConn2 -- I2R/RConn1
  Subsystem/RConn1 -- Iron Loss/LConn1

== system BEVplantModel/Vehicle/Rear Motor (EM2)/Emotor/Sensing Ref Torque ==
  " " : Inport
  Simulink-PS G1 : nesl_utility/Simulink-PS Converter  PhysicalDomain=network_engine_domain  SubClassName=ps_input  LeftPortType=input  RightPortType=output  PseudoPeriodic=off  Frequencies=[]  NoiseDistribution=none  NoiseParameters=[]  Unit=N*m  AffineConversion=off  FilteringAndDerivatives=zero  SimscapeFilterOrder=1  InputFilterTimeConstant=1e-6  UdotUserProvided=1
  "  " : PMIOPort  Side=Right
  wires:
  " "/1 -> Simulink-PS G1/1
  connections:
  Simulink-PS G1/RConn1 -- "  "/RConn1

== system BEVplantModel/Vehicle/Rear Motor (EM2)/Emotor/Sensing wMotor ==
  PS-Simulink Converter : nesl_utility/PS-Simulink Converter  PhysicalDomain=network_engine_domain  SubClassName=ps_output  LeftPortType=input  RightPortType=output  PseudoPeriodic=off  Frequencies=[]  VectorFormat=1-D array  Unit=rpm  AffineConversion=off
  PS : PMIOPort  Side=Left
  SL : Outport  VectorParamsAs1DForOutWhenUnconnected=off
  wires:
  PS-Simulink Converter/1 -> SL/1
  connections:
  PS/RConn1 -- PS-Simulink Converter/LConn1

== system BEVplantModel/Vehicle/Rear Motor (EM2)/Emotor/Speed Measurement ==
  Ideal Rotational Motion Sensor : fl_lib/Mechanical/Mechanical Sensors/Ideal Rotational Motion Sensor  reference=foundation.enum.MeasurementReference.difference  acceleration_port=false  velocity_port=true  position_port=true  wrap_angle=false  offset=0 rad
  MRRef1 : fl_lib/Mechanical/Rotational Elements/Mechanical Rotational Reference
  spd : PMIOPort  Side=Right
  mot : PMIOPort  Port=2  Side=Left
  connections:
  MRRef1/LConn1 -- Ideal Rotational Motion Sensor/RConn1
  mot/RConn1 -- Ideal Rotational Motion Sensor/LConn1
  spd/RConn1 -- Ideal Rotational Motion Sensor/RConn2

== system BEVplantModel/Vehicle/Rear Motor (EM2)/Emotor/Temperature ==
  Rotor Thermal Block : Subsystem
  Stator Thermal Block : Subsystem
  I2R : PMIOPort  Side=Left
  H_rt : PMIOPort  Port=2  Side=Left
  H_st : PMIOPort  Port=3  Side=Left
  HTC_TC : PMIOPort  Port=4  Side=Left
  HTC : PMIOPort  Port=5  Side=Left
  Tc : PMIOPort  Port=6  Side=Right
  Tm : PMIOPort  Port=7  Side=Right
  H : PMIOPort  Port=8  Side=Right
  connections:
  H/RConn1 -- Stator Thermal Block/LConn1
  H_rt/RConn1 -- Rotor Thermal Block/RConn1
  H_st/RConn1 -- Stator Thermal Block/RConn1
  I2R/RConn1 -- Stator Thermal Block/RConn2
  HTC_TC/RConn1 -- Rotor Thermal Block/RConn2
  HTC/RConn1 -- Rotor Thermal Block/RConn3
  Tm/RConn1 -- Rotor Thermal Block/LConn1
  Tc/RConn1 -- Stator Thermal Block/LConn2

== system BEVplantModel/Vehicle/Rear Motor (EM2)/Emotor/current sensing2 ==
  Current Sensor : fl_lib/Electrical/Electrical Sensors/Current Sensor
  " " : PMIOPort  Side=Left
  "  " : PMIOPort  Port=2  Side=Right
  "  I" : PMIOPort  Port=3  Side=Right
  connections:
  Current Sensor/RConn2 -- "  "/RConn1
  Current Sensor/LConn1 -- " "/RConn1
  Current Sensor/RConn1 -- "  I"/RConn1
